simulink model "Single_Phase_Double_Stage_Boost_Converter"  (R2023b)
settings: Solver=ode45  StartTime=0.0  StopTime=0.5  MaxStep=1e-7  MinStep=1e-8  RelTol=1e-3
libraries: spsIGBTDiodeLib x4, spsSeriesRLCBranchLib x4, spsVoltageMeasurementLib x2, spsCurrentMeasurementLib x2, simulink x1, spsDCVoltageSourceLib x1, spspowerguiLib x1, sps_lib x1
settings Model: Creator=aoni5  LastModifiedBy=aoni5

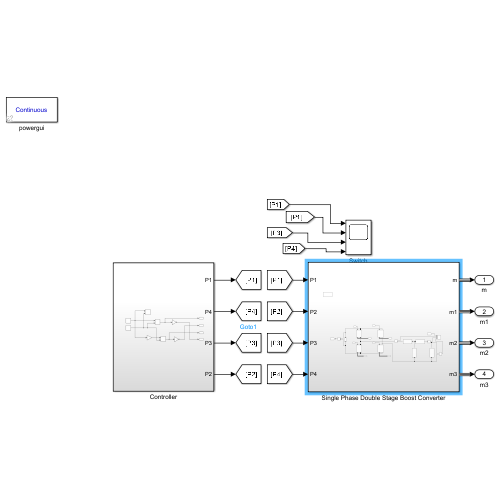
[thumbnail: Simulink's stored preview of the top-level diagram]
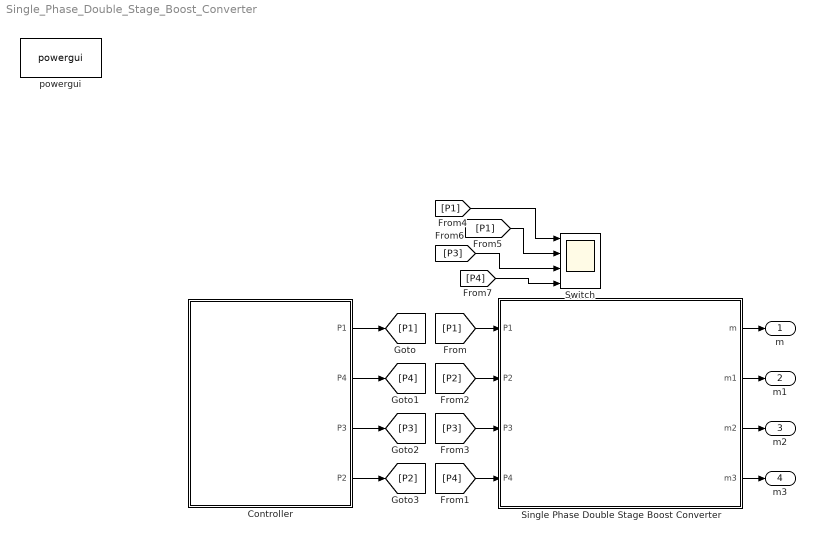
== system Single_Phase_Double_Stage_Boost_Converter ==
  Controller : Subsystem
  Single Phase Double Stage Boost Converter : Subsystem
  Switch : Scope  NumInputPorts=4
  powergui : sps_lib/powergui  Priority=1  SimulationMode=Continuous  SampleTime=50e-6  frequency=60  Iterations=50  frequencyindice=0  Pbase=100e6  ErrMax=1e-4  UnitsV=kV  UnitsW=MW  buscounter=0  FunctionMessages=off  echomessages=off  EnableUseOfTLC=off  CurrentSourceSwitches=off  DisableSnubberDevices=off  DisableRonSwitches=off  DisableVfSwitches=off  DisplayEquations=off  AutomaticDiscreteSolvers=off  SolverType=Tustin/Backward Euler (TBE)  Interpol=off  ExternalGateDelay=off  methode=off  Ts=100  x0status=blocks  SPID=on  SwTol=0  HookPort=off  NonlinearTolerance=1e-4  nMaxIteration=100  ContinueOnMaxIteration=off  RestoreLinks=warning  ResistiveCurrentMeasurement=off  Frange=[0:2:500]  Ylog=off  Xlog=on  ShowGrid=off  save=off  variable=ZData  structure=0  ZoomFFT=off  StartTime=0.0  cycles=1  DisplayStyle=1  fundamental=60  FreqAxis=off  MaxFrequency=1000  frequencyindicesteady=1  RmsSteady=1  display=off
  m : Outport
  m1 : Outport  Port=2
  m2 : Outport  Port=3
  m3 : Outport  Port=4
  wires:
  Controller/2(P4) -> [P4]
  Controller/1(P1) -> [P1]
  Controller/3(P3) -> [P3]
  Controller/4(P2) -> [P2]
  Single Phase Double Stage Boost Converter/1(m) -> m/1
  Single Phase Double Stage Boost Converter/2(m1) -> m1/1
  Single Phase Double Stage Boost Converter/3(m2) -> m2/1
  Single Phase Double Stage Boost Converter/4(m3) -> m3/1
  [P1] -> Single Phase Double Stage Boost Converter/1(P1)
  [P4] -> Single Phase Double Stage Boost Converter/4(P4)
  [P3] -> Single Phase Double Stage Boost Converter/3(P3)
  [P2] -> Single Phase Double Stage Boost Converter/2(P2)
  [P1] -> Switch/1
  [P1] -> Switch/2
  [P3] -> Switch/3
  [P4] -> Switch/4

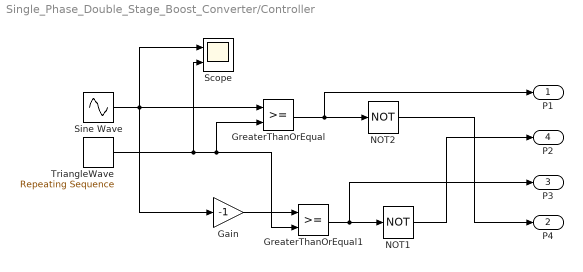
== system Single_Phase_Double_Stage_Boost_Converter/Controller ==
  Gain : Gain  Gain=-1
  GreaterThanOrEqual : RelationalOperator  OutDataTypeStr=boolean  RndMeth=Simplest  InputSameDT=off
  GreaterThanOrEqual1 : RelationalOperator  OutDataTypeStr=boolean  RndMeth=Simplest  InputSameDT=off
  NOT1 : Logic  Operator=NOT  IconShape=distinctive  AllPortsSameDT=off  OutDataTypeStr=boolean
  NOT2 : Logic  Operator=NOT  IconShape=distinctive  AllPortsSameDT=off  OutDataTypeStr=boolean
  Scope : Scope  NumInputPorts=2
  Sine Wave : Sin  Amplitude=0.5  Frequency=2*pi*60  SampleTime=5e-7
  TriangleWave : simulink/Sources/Repeating Sequence  rep_seq_t=[0 50e-6 100e-6]  rep_seq_y=[-1 0 1]
  P1 : Outport
  P4 : Outport  Port=2
  P3 : Outport  Port=3
  P2 : Outport  Port=4
  wires:
  NOT1/1 -> P2/1
  GreaterThanOrEqual/1 -> P1/1, NOT2/1
  TriangleWave/1 -> GreaterThanOrEqual1/2, GreaterThanOrEqual/2, Scope/2
  Sine Wave/1 -> Gain/1, Scope/1, GreaterThanOrEqual/1
  Gain/1 -> GreaterThanOrEqual1/1
  GreaterThanOrEqual1/1 -> P3/1, NOT1/1
  NOT2/1 -> P4/1

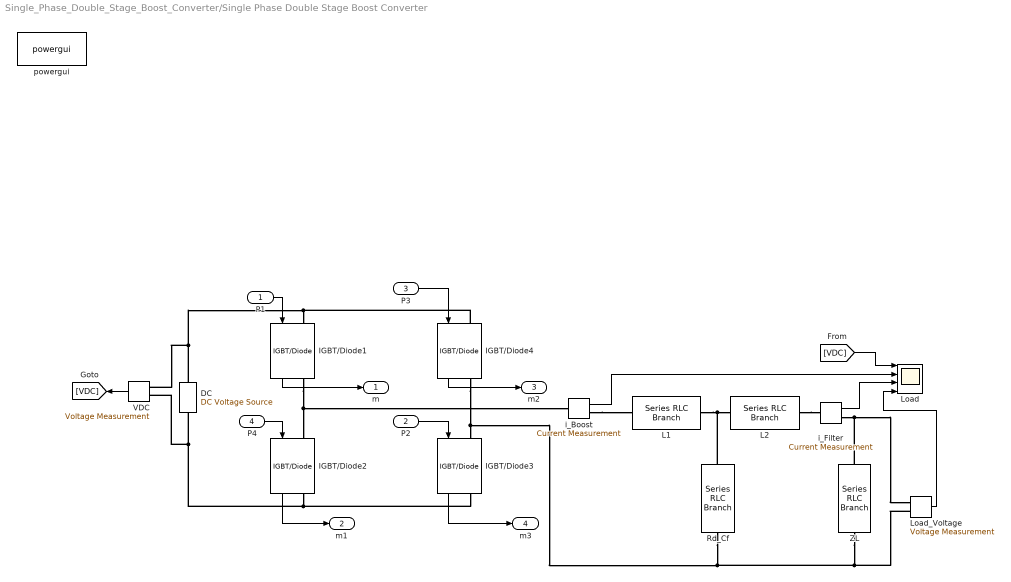
== system Single_Phase_Double_Stage_Boost_Converter/Single Phase Double Stage Boost Converter ==
  P1 : Inport
  P2 : Inport  Port=2
  P3 : Inport  Port=3
  P4 : Inport  Port=4
  DC : spsDCVoltageSourceLib/DC Voltage Source  Amplitude=300  Measurements=None
  IGBT/Diode{1..4} (4 alike) : spsIGBTDiodeLib/IGBT//Diode  Ron=1e-3  Rs=1e5  Cs=inf  Measurements=on
  L1 : spsSeriesRLCBranchLib/Series RLC Branch  LConnTagsString=__new0  RConnTagsString=__new0  BranchType=L  Resistance=2.5  Inductance=1e-3  SetiL0=off  InitialCurrent=0  Capacitance=50e-6  Setx0=off  InitialVoltage=0  Measurements=None
  L2 : spsSeriesRLCBranchLib/Series RLC Branch  LConnTagsString=__new0  RConnTagsString=__new0  BranchType=L  Resistance=2.5  Inductance=250e-6  SetiL0=off  InitialCurrent=0  Capacitance=50e-6  Setx0=off  InitialVoltage=0  Measurements=None
  Load : Scope  NumInputPorts=4
  Load_Voltage : spsVoltageMeasurementLib/Voltage Measurement  PhasorSimulation=off  OutputType=Complex  PSBequivalent=0
  Rd_Cf : spsSeriesRLCBranchLib/Series RLC Branch  LConnTagsString=__new0  RConnTagsString=__new0  BranchType=RC  Resistance=5.97  Inductance=1e-3  SetiL0=off  InitialCurrent=0  Capacitance=5.6e-6  Setx0=off  InitialVoltage=0  Measurements=None
  VDC : spsVoltageMeasurementLib/Voltage Measurement  PhasorSimulation=off  OutputType=Complex  PSBequivalent=0
  ZL : spsSeriesRLCBranchLib/Series RLC Branch  LConnTagsString=__new0  RConnTagsString=__new0  BranchType=RL  Resistance=5  Inductance=5e-3  SetiL0=off  InitialCurrent=0  Capacitance=1e-6  Setx0=off  InitialVoltage=0  Measurements=None
  i_Boost : spsCurrentMeasurementLib/Current Measurement  PhasorSimulation=off  OutputType=Complex  PSBequivalent=0
  i_Filter : spsCurrentMeasurementLib/Current Measurement  PhasorSimulation=off  OutputType=Complex  PSBequivalent=0
  powergui : spspowerguiLib/powergui  Priority=1  SimulationMode=Continuous  SampleTime=50e-6  frequency=60  Iterations=50  frequencyindice=60  Pbase=100e6  ErrMax=1e-4  UnitsV=kV  UnitsW=MW  buscounter=0  FunctionMessages=off  echomessages=off  EnableUseOfTLC=off  CurrentSourceSwitches=off  DisableSnubberDevices=off  DisableRonSwitches=off  DisableVfSwitches=off  DisplayEquations=off  AutomaticDiscreteSolvers=off  SolverType=Tustin/Backward Euler (TBE)  Interpol=off  ExternalGateDelay=off  methode=off  Ts=100  x0status=blocks  SPID=on  SwTol=0  HookPort=off  NonlinearTolerance=1e-4  nMaxIteration=100  ContinueOnMaxIteration=off  RestoreLinks=warning  ResistiveCurrentMeasurement=off  Frange=[0:2:500]  Ylog=off  Xlog=on  ShowGrid=off  save=off  variable=ZData  structure=0  ZoomFFT=off  StartTime=0.0  cycles=1  DisplayStyle=1  fundamental=60  FreqAxis=off  MaxFrequency=1000  frequencyindicesteady=1  RmsSteady=1  display=off
  m : Outport
  m1 : Outport  Port=2
  m2 : Outport  Port=3
  m3 : Outport  Port=4
  wires:
  P3/1 -> IGBT/Diode4/1
  IGBT/Diode1/1 -> m/1
  IGBT/Diode2/1 -> m1/1
  P1/1 -> IGBT/Diode1/1
  P4/1 -> IGBT/Diode2/1
  P2/1 -> IGBT/Diode3/1
  IGBT/Diode4/1 -> m2/1
  IGBT/Diode3/1 -> m3/1
  i_Boost/1 -> Load/2
  Load_Voltage/1 -> Load/4
  i_Filter/1 -> Load/3
  VDC/1 -> [VDC]
  [VDC] -> Load/1
  connections:
  IGBT/Diode1/LConn1 -- VDC/LConn1 -- DC/RConn1 -- IGBT/Diode4/LConn1
  IGBT/Diode2/RConn1 -- IGBT/Diode3/RConn1 -- VDC/LConn2 -- DC/LConn1
  Rd_Cf/RConn1 -- L1/RConn1 -- L2/LConn1
  IGBT/Diode4/RConn1 -- Load_Voltage/LConn2 -- ZL/LConn1 -- Rd_Cf/LConn1 -- IGBT/Diode3/LConn1
  IGBT/Diode1/RConn1 -- i_Boost/LConn1 -- IGBT/Diode2/LConn1
  i_Boost/RConn1 -- L1/LConn1
  ZL/RConn1 -- i_Filter/RConn1 -- Load_Voltage/LConn1
  L2/RConn1 -- i_Filter/LConn1
